simulink model "buck_bode_plot"  (R2023b)
settings: Solver=VariableStepAuto  StartTime=0.0  StopTime=Tend  RelTol=1e-3
values from neighbouring files (symbols this model uses):
  Cdc = 1e-4    (= 0.0001)    [DE_DEMO2.m]
  Ki = DE_out.best_sol(1,2,end)    [DE_DEMO2.m]    (also in MO_DEMO_BUCK.m = x(1,2))
  Kp = DE_out.best_sol(1,1,end)    [DE_DEMO2.m]    (also in MO_DEMO_BUCK.m = x(1,1))
  L = 1e-4    (= 0.0001)    [DE_DEMO2.m]
  Ro = 1    [DE_DEMO2.m]
  Tend = Ts*1000    (= 0.1)    [DE_DEMO2.m]
  Ts = 1/Fs    (= 0.0001)    [DE_DEMO2.m]
  Tsamp = 1/Fsamp    (= 1e-06)    [DE_DEMO2.m]
  Ttrig = (Tstart+Tend)/2    (= 0.075)    [DE_DEMO2.m]
  Vg = 100    [DE_DEMO2.m]
  Vref1 = 40    [DE_DEMO2.m]
  Vref2 = 60    [DE_DEMO2.m]
libraries: spsSeriesRLCBranchLib x3, spsMosfetLib x2, slctrl_linear x1, simulink x1, spsCurrentMeasurementLib x1, spsDCVoltageSourceLib x1, spsVoltageMeasurementLib x1, simulink_extras x1, sps_lib x1
settings Model: Creator=Hyeongmeen  LastModifiedBy=baik3-ad

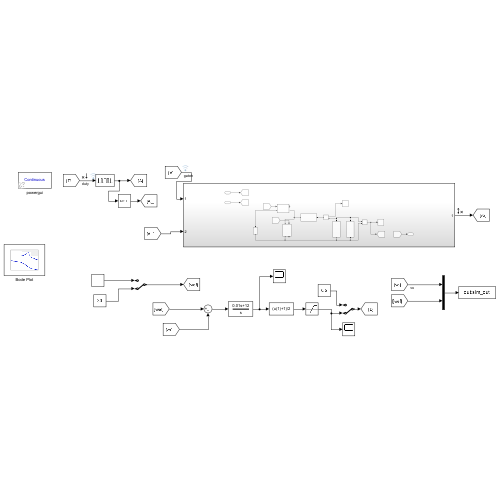
[thumbnail: Simulink's stored preview of the top-level diagram]
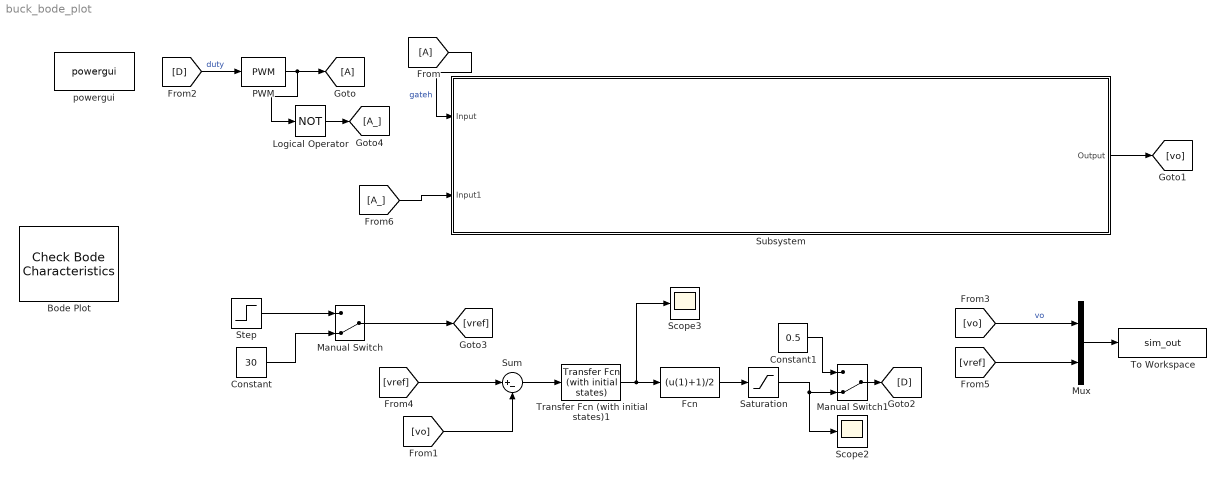
== system buck_bode_plot ==
  Bode Plot : slctrl_linear/Check Bode  Characteristics  InstantiateOnLoad=on  SaveOperatingPoints=off  LinearizationIOs={'/Subsystem', 1, 'out', 'on', '';'/From2', 1, 'in', 'on', ''}  LinearizeAt=SnapshotTimes  SnapshotTimes=[0 Tend]  TriggerType=rising  SampleTime=auto  RateConversionMethod=zoh  PreWarpFreq=10  UseExactDelayModel=off  UseFullBlockNameLabels=on  UseBusSignalLabels=on  enabled=on  stopWhenAssertionFail=off  export=off  ViewDlgPos=[267 201 802 565]  OpenViewOnLoad=off  LaunchViewOnOpen=off  FrequencyUnits=rad/s  MagnitudeUnits=dB  PhaseUnits=deg  TimeUnits=seconds  EnableUpperBound=off  UpperBoundFrequencies=[]  UpperBoundMagnitudes=[]  EnableLowerBound=off  LowerBoundFrequencies=[]  LowerBoundMagnitudes=[]
      settings: LibrarySourceBlock=slctrlblks/Linear Analysis Plots/Bode Plot  SaveToWorkspace=on  SaveName=sys
  Constant : Constant  Value=30
  Constant1 : Constant  Value=0.5
  Fcn : Fcn  Expr=(u(1)+1)/2
  From : From
  Goto : Goto
  Logical Operator : Logic  Operator=NOT  AllPortsSameDT=off  OutDataTypeStr=boolean
  Manual Switch : ManualSwitch  CurrentSetting=0
  Manual Switch1 : ManualSwitch  CurrentSetting=0
  Mux : Mux  Inputs=2
  PWM : simulink/Discontinuities/PWM  DisableCoverage=on  Period=Ts  InitialDelay=0  DisallowZeroDutyCycle=off  RunAtFixedTimeIntervals=off  SampleTime=0.1
  Saturation : Saturate  UpperLimit=1  LowerLimit=0
  Scope2 : Scope
  Scope3 : Scope
  Step : Step  Time=Ttrig  Before=Vref1  After=Vref2  SampleTime=Tsamp
  Subsystem : Subsystem
  Sum : Sum  Inputs=|+-
  To Workspace : ToWorkspace  VariableName=sim_out  SaveFormat=Timeseries  SampleTime=Tsamp
  Transfer Fcn (with initial states)1 : simulink_extras/Additional Linear/Transfer Fcn (with initial states)  N=[Kp Ki]  D="[1  0]"  X0=0
  powergui : sps_lib/powergui  Priority=1  SimulationMode=Continuous  SampleTime=Tsamp  frequency=60  Iterations=50  frequencyindice=0  Pbase=100e6  ErrMax=1e-4  UnitsV=kV  UnitsW=MW  buscounter=0  FunctionMessages=off  echomessages=off  EnableUseOfTLC=off  CurrentSourceSwitches=off  DisableSnubberDevices=off  DisableRonSwitches=off  DisableVfSwitches=off  DisplayEquations=off  AutomaticDiscreteSolvers=off  SolverType=Tustin/Backward Euler (TBE)  Interpol=off  ExternalGateDelay=off  methode=off  Ts=100  x0status=blocks  SPID=on  SwTol=0  HookPort=off  NonlinearTolerance=1e-4  nMaxIteration=100  ContinueOnMaxIteration=off  RestoreLinks=warning  ResistiveCurrentMeasurement=off  Frange=[0:2:500]  Ylog=off  Xlog=on  ShowGrid=off  save=off  variable=ZData  structure=0  ZoomFFT=off  StartTime=0.0  cycles=1  DisplayStyle=1  fundamental=60  FreqAxis=off  MaxFrequency=1000  frequencyindicesteady=1  RmsSteady=1  display=off
  wires:
  PWM/1 -> Logical Operator/1, Goto/1
  [D] -> PWM/1  "duty"
  [vref] -> Sum/1
  [vo] -> Sum/2
  Sum/1 -> Transfer Fcn (with initial states)1/1
  Transfer Fcn (with initial states)1/1 -> Scope3/1, Fcn/1
  Fcn/1 -> Saturation/1
  Manual Switch/1 -> [vref]
  [vo] -> Mux/1  "vo"
  [vref] -> Mux/2
  Mux/1 -> To Workspace/1
  Saturation/1 -> Manual Switch1/2, Scope2/1
  Logical Operator/1 -> [A_]
  From/1 -> Subsystem/1(Input)  "gateh"
  [A_] -> Subsystem/2(Input1)
  Subsystem/1(Output) -> [vo]
  Step/1 -> Manual Switch/1
  Constant/1 -> Manual Switch/2
  Manual Switch1/1 -> [D]
  Constant1/1 -> Manual Switch1/1

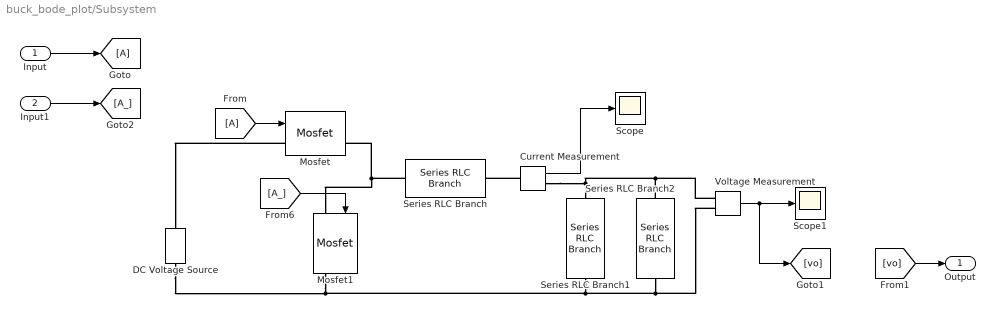
== system buck_bode_plot/Subsystem ==
  Input : Inport
  Input1 : Inport  Port=2
  Current Measurement : spsCurrentMeasurementLib/Current Measurement  PhasorSimulation=off  OutputType=Complex  PSBequivalent=0
  DC Voltage Source : spsDCVoltageSourceLib/DC Voltage Source  Amplitude=Vg  Measurements=None
  From : From
  Goto : Goto
  Mosfet : spsMosfetLib/Mosfet  Ron=Rdson  Lon=0  Rd=Rdson  Vfd=0  IC=0  Rs=1e5  Cs=inf  Measurements=on
  Mosfet1 : spsMosfetLib/Mosfet  Ron=Rdson  Lon=0  Rd=Rdson  Vfd=0  IC=0  Rs=1e5  Cs=inf  Measurements=on
  Scope : Scope
  Scope1 : Scope
  Series RLC Branch : spsSeriesRLCBranchLib/Series RLC Branch  LConnTagsString=__new0  RConnTagsString=__new0  BranchType=L  Resistance=1  Inductance=L  SetiL0=off  InitialCurrent=0  Capacitance=1e-6  Setx0=off  InitialVoltage=0  Measurements=None
  Series RLC Branch1 : spsSeriesRLCBranchLib/Series RLC Branch  LConnTagsString=__new0  RConnTagsString=__new0  BranchType=C  Resistance=1  Inductance=1e-3  SetiL0=off  InitialCurrent=0  Capacitance=Cdc  Setx0=off  InitialVoltage=0  Measurements=None
  Series RLC Branch2 : spsSeriesRLCBranchLib/Series RLC Branch  LConnTagsString=__new0  RConnTagsString=__new0  BranchType=R  Resistance=Ro  Inductance=1e-3  SetiL0=off  InitialCurrent=0  Capacitance=1e-6  Setx0=off  InitialVoltage=0  Measurements=None
  Voltage Measurement : spsVoltageMeasurementLib/Voltage Measurement  PhasorSimulation=off  OutputType=Complex  PSBequivalent=0
  Output : Outport
  wires:
  Current Measurement/1 -> Scope/1
  Voltage Measurement/1 -> [vo], Scope1/1
  From/1 -> Mosfet/1
  [A_] -> Mosfet1/1
  Input/1 -> Goto/1
  Input1/1 -> [A_]
  [vo] -> Output/1
  connections:
  Series RLC Branch1/RConn1 -- Voltage Measurement/LConn2 -- Series RLC Branch2/RConn1 -- Mosfet1/RConn1 -- DC Voltage Source/LConn1
  Series RLC Branch1/LConn1 -- Series RLC Branch2/LConn1 -- Voltage Measurement/LConn1 -- Current Measurement/RConn1
  Mosfet/RConn1 -- Mosfet1/LConn1 -- Series RLC Branch/LConn1
  Mosfet/LConn1 -- DC Voltage Source/RConn1
  Current Measurement/LConn1 -- Series RLC Branch/RConn1
